simulink model "torque_controller_subsystem_completed_V2_R2019"  (R2019a)
settings: Solver=VariableStepAuto  StartTime=0.0  StopTime=5  RelTol=1e-3
model workspace (MAT data in the model file):
  DCBusVoltage = 24
  K_e = 221.0633
  L_d = 0.003482
  L_q = 0.00456
  Machine_Temperature = 25
  N = 9
  Peak_Current_String = 'Peak Current = 6.000000'
  PhaseAdvancesPerCycle = 36
  Phase_Advance_String = 'PhaseAdvance = 180.000000'
  PointsPerCycle = 36
  Rload = 1000000
  Rs = 0.624570538244
  Shaft_Speed = 27
  MCOS : class17 (value not decoded)
  MCOS : class17 (value not decoded)
  angleVec = [0 1.11111111111 2.22222222222 3.33333333333 4.44444444444 5.55555555556 6.66666666667 7.77777777778 8.88888888889 10 11.1111111111 12.2222222222 ... (37 elements, 1x37)]
  dq_inductance = 0.008366
  fluxAmat = [5.78758604472e-05 -0.00245230641441 -0.00496086974489 -0.00746825845512 -0.00997085180846 -0.0124701917234 -0.0149650380151 -0.0174527751443 -0.0199339133996 -0.0224017046643 -0.0248570910938 -0.0273006981398 ... (16428 elements, 12x37x37)]
  fluxD = 0.129208614948
  fluxDmat = [0.129332720835 0.129331856309 0.129330386347 0.129326055027 0.129320008491 0.129311398581 0.12929964601 0.129284600324 0.129267743431 0.129250546721 0.129230887735 0.129208614948 ... (16428 elements, 12x37x37)]
  fluxQ = -0.0273006981398
  fluxQmat = [5.78758604472e-05 -0.00245230641441 -0.00496086974489 -0.00746825845512 -0.00997085180846 -0.0124701917234 -0.0149650380151 -0.0174527751443 -0.0199339133996 -0.0224017046643 -0.0248570910938 -0.0273006981398 ... (16428 elements, 12x37x37)]
  fluxes = [-0.0273006981398; -0.0982475938625; 0.125548292002]
  funcresult = 0
  gammaVec = [-180 -170 -160 -150 -140 -130 -120 -110 -100 -90 -80 -70 ... (37 elements, 1x37)]
  i = 12
  invP = [-2.44929359829e-16  1; -0.866025403784  -0.5; 0.866025403784  -0.5]
  j = 37
  m = 37
  magVec = [0 0.545454545455 1.09090909091 1.63636363636 2.18181818182 2.72727272727 3.27272727273 3.81818181818 4.36363636364 4.90909090909 5.45454545455 6]
  nGamma = 37
  nMag = 12
  nX = 37
  poleNumber = 18
  pole_pairs = 9
  res1 = 0
  res2 = 0
  res3 = 0
  resistance_per_phase = 0.6246
  torque = -10.6713070894
  torqueMat = [-0.000127780443833 -0.972425785337 -1.94471415001 -2.91686171491 -3.8887574387 -4.86000619896 -5.83073162472 -6.80075888771 -7.77012767412 -8.7384579087 -9.70556312381 -10.6713070894 ... (16428 elements, 12x37x37)]
  torque_constant = 1.7505
  x1 = 360
  x2 = 360
  x3 = 360
  xe = 6.28318530718
  xlabel_string = 'Rotor angle (electrical °)'
  ylabel_string = 'Phase advance (°)'
libraries: fl_lib x12, nesl_utility x12, ee_lib x8, eeTransforms x3, simulink x2, powerlib_meascontrol x1
(part 2 of 2)

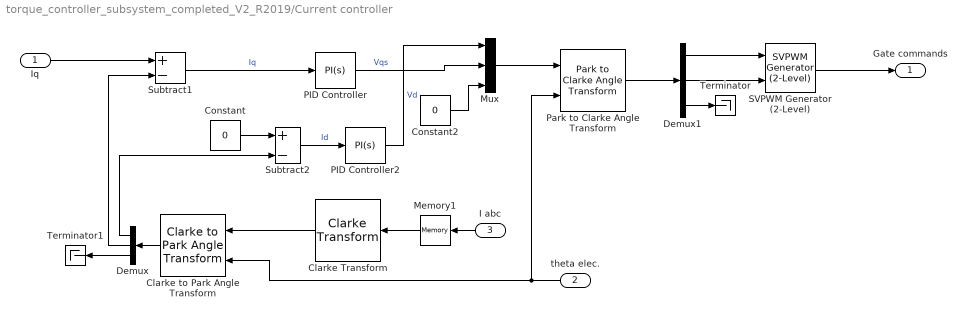
== system torque_controller_subsystem_completed_V2_R2019/Current controller ==
  Iq : Inport
  theta elec. : Inport  Port=2
  I abc : Inport  Port=3
  Clarke Transform : eeTransforms/Clarke Transform  PowerInvariant=off
      settings: SourceProductBaseCode=PS
  Clarke to Park Angle Transform : eeTransforms/Clarke to Park Angle Transform  AxisAlignment=D-axis
      settings: SourceProductBaseCode=PS
  Constant : Constant  Value=0
  Constant2 : Constant  Value=0
  Demux : Demux  Outputs=3
  Demux1 : Demux  Outputs=3
  Memory1 : Memory
  Mux : Mux  Inputs=3
  PID Controller : simulink/Continuous/PID Controller  Controller=PI  Form=Parallel  TimeDomain=Continuous-time  SampleTime=-1  IntegratorMethod=Forward Euler  FilterMethod=Forward Euler  ControllerParametersSource=internal  P=0.23449  I=72.7938  D=0  UseFilter=on  N=100  TunerSelectOption=Transfer Function Based (PID Tuner App)  InitialConditionSource=internal  InitialConditionForIntegrator=0  InitialConditionForFilter=0  DifferentiatorICPrevScaledInput=0  ExternalReset=none  TrackingMode=off  Kt=1  LimitOutput=off  UpperSaturationLimit=inf  LowerSaturationLimit=-inf  LinearizeAsGain=on  AntiWindupMode=none  Kb=1  POutMin=[]  POutMax=[]  IOutMin=[]  IOutMax=[]  DOutMin=[]  DOutMax=[]  NOutMin=[]  NOutMax=[]  SumOutMin=[]  SumOutMax=[]  SaturationOutMin=[]  SaturationOutMax=[]  PParamMin=[]  PParamMax=[]  IParamMin=[]  IParamMax=[]  DParamMin=[]  DParamMax=[]  NParamMin=[]  NParamMax=[]  KbParamMin=[]  KbParamMax=[]  KtParamMin=[]  KtParamMax=[]  KbOutMin=[]  KbOutMax=[]  KtOutMin=[]  KtOutMax=[]  IntegratorOutMin=[]  IntegratorOutMax=[]  FilterOutMin=[]  FilterOutMax=[]  SumI1OutMin=[]  SumI1OutMax=[]  SumI2OutMin=[]  SumI2OutMax=[]  SumI3OutMin=[]  SumI3OutMax=[]  SumI4OutMin=[]  SumI4OutMax=[]  SumDOutMin=[]  SumDOutMax=[]  DifferentiatorOutMin=[]  DifferentiatorOutMax=[]  FilterDiffOutCoefMin=[]  FilterDiffOutCoefMax=[]  ReciprocalOutMin=[]  ReciprocalOutMax=[]  SumDenOutMin=[]  SumDenOutMax=[]  SumNumOutMin=[]  SumNumOutMax=[]  DivideOutMin=[]  DivideOutMax=[]  IntegratorContinuousStateAttributes=''  IntegratorStateMustResolveToSignalObject=off  IntegratorRTWStateStorageClass=Auto  FilterContinuousStateAttributes=''  FilterStateMustResolveToSignalObject=off  FilterRTWStateStorageClass=Auto  ParallelPVariant=InternalParameters  IdealPVariant=Disabled  IVariant=InternalParameters  DVariant=Disabled  IntegratorVariant=Continuous  SatVariant=Disabled  AWVariant=Passthrough  PCopyVariant=Disabled  TRVariant=Disabled  FdbkBlocksVariant=Forward  IdealPFdbkVariant=Disabled  SatFdbkVariant=Disabled  DerivativeFilterVariant=Disabled  NVariant=Disabled  NCopyVariant=Disabled_SignalSpec  FilterICVariant=Disabled  IntegratorICVariant=InternalICs  ExternalResetVariant=Disabled  TRSumVariant=Passthrough  SumFdbkVariant=Disabled  SumVariant=Sum_PI
  PID Controller2 : simulink/Continuous/PID Controller  Controller=PI  Form=Parallel  TimeDomain=Continuous-time  SampleTime=-1  IntegratorMethod=Forward Euler  FilterMethod=Forward Euler  ControllerParametersSource=internal  P=0.17425  I=69.1084  D=0  UseFilter=on  N=100  TunerSelectOption=Transfer Function Based (PID Tuner App)  InitialConditionSource=internal  InitialConditionForIntegrator=0  InitialConditionForFilter=0  DifferentiatorICPrevScaledInput=0  ExternalReset=none  TrackingMode=off  Kt=1  LimitOutput=off  UpperSaturationLimit=inf  LowerSaturationLimit=-inf  LinearizeAsGain=on  AntiWindupMode=none  Kb=1  POutMin=[]  POutMax=[]  IOutMin=[]  IOutMax=[]  DOutMin=[]  DOutMax=[]  NOutMin=[]  NOutMax=[]  SumOutMin=[]  SumOutMax=[]  SaturationOutMin=[]  SaturationOutMax=[]  PParamMin=[]  PParamMax=[]  IParamMin=[]  IParamMax=[]  DParamMin=[]  DParamMax=[]  NParamMin=[]  NParamMax=[]  KbParamMin=[]  KbParamMax=[]  KtParamMin=[]  KtParamMax=[]  KbOutMin=[]  KbOutMax=[]  KtOutMin=[]  KtOutMax=[]  IntegratorOutMin=[]  IntegratorOutMax=[]  FilterOutMin=[]  FilterOutMax=[]  SumI1OutMin=[]  SumI1OutMax=[]  SumI2OutMin=[]  SumI2OutMax=[]  SumI3OutMin=[]  SumI3OutMax=[]  SumI4OutMin=[]  SumI4OutMax=[]  SumDOutMin=[]  SumDOutMax=[]  DifferentiatorOutMin=[]  DifferentiatorOutMax=[]  FilterDiffOutCoefMin=[]  FilterDiffOutCoefMax=[]  ReciprocalOutMin=[]  ReciprocalOutMax=[]  SumDenOutMin=[]  SumDenOutMax=[]  SumNumOutMin=[]  SumNumOutMax=[]  DivideOutMin=[]  DivideOutMax=[]  IntegratorContinuousStateAttributes=''  IntegratorStateMustResolveToSignalObject=off  IntegratorRTWStateStorageClass=Auto  FilterContinuousStateAttributes=''  FilterStateMustResolveToSignalObject=off  FilterRTWStateStorageClass=Auto  ParallelPVariant=InternalParameters  IdealPVariant=Disabled  IVariant=InternalParameters  DVariant=Disabled  IntegratorVariant=Continuous  SatVariant=Disabled  AWVariant=Passthrough  PCopyVariant=Disabled  TRVariant=Disabled  FdbkBlocksVariant=Forward  IdealPFdbkVariant=Disabled  SatFdbkVariant=Disabled  DerivativeFilterVariant=Disabled  NVariant=Disabled  NCopyVariant=Disabled_SignalSpec  FilterICVariant=Disabled  IntegratorICVariant=InternalICs  ExternalResetVariant=Disabled  TRSumVariant=Passthrough  SumFdbkVariant=Disabled  SumVariant=Sum_PI
  Park to Clarke Angle Transform : eeTransforms/Park to Clarke Angle Transform  AxisAlignment=D-axis
      settings: SourceProductBaseCode=PS
  SVPWM Generator (2-Level) : powerlib_meascontrol/Pulse & Signal Generators/SVPWM Generator (2-Level)  InputType=alpha-beta components  SwitchingPattern=Pattern #1  Fc=2000  ParUref=[0.8 -30 50]  Ts=0
      settings: SourceProductBaseCode=PS
  Subtract1 : Sum  Inputs=+-
  Subtract2 : Sum  Inputs=+-
  Terminator : Terminator
  Terminator1 : Terminator
  Gate commands : Outport
  wires:
  theta elec./1 -> Clarke to Park Angle Transform/2, Park to Clarke Angle Transform/2
  Subtract1/1 -> PID Controller/1  "Iq"
  Demux1/1 -> SVPWM Generator (2-Level)/1
  Mux/1 -> Park to Clarke Angle Transform/1
  PID Controller/1 -> Mux/2  "Vqs"
  Demux1/2 -> SVPWM Generator (2-Level)/2
  Clarke Transform/1 -> Clarke to Park Angle Transform/1
  Subtract2/1 -> PID Controller2/1  "Id"
  Demux/1 -> Subtract2/2
  Clarke to Park Angle Transform/1 -> Demux/1
  Demux1/3 -> Terminator/1
  Demux/2 -> Subtract1/2
  Constant2/1 -> Mux/3
  Demux/3 -> Terminator1/1
  Park to Clarke Angle Transform/1 -> Demux1/1
  Constant/1 -> Subtract2/1
  Memory1/1 -> Clarke Transform/1
  PID Controller2/1 -> Mux/1  "Vd"
  SVPWM Generator (2-Level)/1 -> Gate commands/1
  Iq/1 -> Subtract1/1
  I abc/1 -> Memory1/1

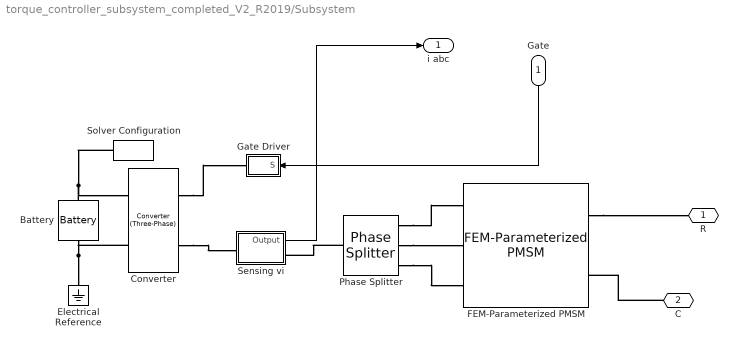
== system torque_controller_subsystem_completed_V2_R2019/Subsystem ==
  Gate : Inport
  Battery : ee_lib/Sources/Battery  Vnom=24 V  R1=2 Ohm  prm_AH=1  AH=50 hr*A  V1=11.5 V  AH1=25 hr*A  prm_R2=1  R2=2000 Ohm  prm_dyn=1  Rp1=0.005 Ohm  tau1=30 s  Rp2=0.005 Ohm  tau2=30 s  Rp3=0.005 Ohm  tau3=30 s  Rp4=0.005 Ohm  tau4=30 s  Rp5=0.005 Ohm  tau5=30 s  prm_fade=1  N_fade=100  AH_fade=45 hr*A  R1_fade=2.02 Ohm  V1_fade=10.35 V  i_specify=off  i_priority=None  i=0 A  i_nominal_specify=off  i_nominal_unit=A  i_nominal_value=1  v_specify=off  v_priority=None  v=0 V  v_nominal_specify=off  v_nominal_unit=V  v_nominal_value=1  charge_specify=off  charge_priority=High  charge=50 hr*A  charge_nominal_specify=off  charge_nominal_unit=hr*A  charge_nominal_value=1  num_cycles_specify=off  num_cycles_priority=High  num_cycles=0  num_cycles_nominal_specify=off  num_cycles_nominal_unit=1  num_cycles_nominal_value=1  thermal_mass=30000 J/K  Tmeas=298.15 K  Vnom_T2=12 V  R1_T2=2.2 Ohm  V1_T2=11.4 V  R2_T2=2200 Ohm  Rp1_T2=0.005 Ohm  tau1_T2=30 s  Rp2_T2=0.005 Ohm  tau2_T2=30 s  Rp3_T2=0.005 Ohm  tau3_T2=30 s  Rp4_T2=0.005 Ohm  tau4_T2=30 s  Rp5_T2=0.005 Ohm  tau5_T2=30 s  Tmeas2=273.15 K  temperature_specify=off  temperature_priority=High  temperature=298.15 K  temperature_nominal_specify=off  temperature_nominal_unit=K  temperature_nominal_value=1
  Converter : ee_lib/Semiconductors & Converters/Converters/Converter (Three-Phase)  device_type=ee.enum.converters.switchingdevice.mosfet  Vf=0.8 V  Ron=17.5*10^-3 Ohm  Rds=17.5 * 10^-3 Ohm  Goff=1e-5 1/Ohm  Vth=0.5 V  Vgt=1 V  Vgt_off=-1 V  Ih=1 A  diode_param=ee.enum.converters.protectiondiode.nodynamics  diode_Vf=0.8 V  diode_Ron=0.001 Ohm  diode_Goff=1e-5 1/Ohm  diode_C=50 nF  diode_iRM=-235 A  diode_iF=300 A  diode_idot=-50 A/us  diode_trr_param=ee.enum.converters.diodetrr.trr_factor  diode_trr_factor=3  diode_trr=15 us  diode_Qrr=1.5e+3 s*uA  snubber_type=ee.enum.converters.snubber.exclude  Rs=0.1 Ohm  Cs=1e-7 F
      settings: SourceProductBaseCode=PS
  Electrical Reference : fl_lib/Electrical/Electrical Elements/Electrical Reference
      settings: SourceProductBaseCode=MT,SS
  FEM-Parameterized PMSM : ee_lib/Electromechanical/Permanent Magnet/FEM-Parameterized PMSM  parameterization=1  winding_type=ee.enum.statorconnection.wye  iVec=[-2, 0, 2] A  xVec=[0, 20, 40, 60] deg  dfluxdiMatrix=0.0002 * ones(3, 4) Wb/A  dfluxdxMatrix=[0, -.16, .16, 0; 0, -.16, .16, 0; 0, -.16, .16, 0] Wb/rad  calculate_torque_matrix=1  TorqueMatrix=zeros(3, 3, 3, 4) N*m  idVec1=[-200, 0, 200] A  iqVec1=[-200, 0, 200] A  LdMatrix=0.0002 * ones(3, 3) H  LqMatrix=0.0002 * ones(3, 3) H  PmMatrix=0.1 * ones(3, 3) Wb  N=6  interp_method=simscape.enum.interpolation.linear  Rs=Rs Ohm  Ms=0.00002 H  losses_oc=[0, 0, 0] W  losses_sc=[0, 0, 0] W  f_losses=140 Hz  Isc_losses=95 A  Inertia=0 kg*m^2  lam=0 N*m/(rad/s)  i_d_specify=off  i_d_priority=High  i_d=0 A  i_d_nominal_specify=off  i_d_nominal_unit=A  i_d_nominal_value=1  i_q_specify=off  i_q_priority=High  i_q=0 A  i_q_nominal_specify=off  i_q_nominal_unit=A  i_q_nominal_value=1  torque_specify=off  torque_priority=None  torque=0 N*m  torque_nominal_specify=off  torque_nominal_unit=N*m  torque_nominal_value=1  angular_velocity_specify=on  angular_velocity_priority=High  angular_velocity=0 rpm  angular_velocity_nominal_specify=off  angular_velocity_nominal_unit=rpm  angular_velocity_nominal_value=1  angular_position_specify=on  angular_position_priority=High  angular_position=0 deg  angular_position_nominal_specify=off  angular_position_nominal_unit=deg  angular_position_nominal_value=1  Tmeas=298.15 K  alpha=3.93e-3 1/K  alpha_flux=-0.001 1/K  stator_thermal_mass=100 J/K  stator_initial_temperatures=[298.15, 298.15, 298.15] K  rotor_thermal_mass=200 J/K  rotor_initial_temperature=298.15 K  Rm_percent_rotor=90  Rd_percent_rotor=30  idVec=[-200, 0, 200] A  iqVec=[-200, 0, 200] A  dfluxAdiaMatrix3D=zeros(3, 3, 4) Wb/A  dfluxAdibMatrix3D=zeros(3, 3, 4) Wb/A  dfluxAdicMatrix3D=zeros(3, 3, 4) Wb/A  dfluxAdxMatrix3D=zeros(3, 3, 4) Wb/rad  TorqueMatrix3D=zeros(3, 3, 4) N*m  iaVec=[-200, 0, 200] A  ibVec=[-200, 0, 200] A  icVec=[-200, 0, 200] A  dfluxAdiaMatrix=zeros(3, 3, 3, 4) Wb/A  dfluxAdibMatrix=zeros(3, 3, 3, 4) Wb/A  dfluxAdicMatrix=zeros(3, 3, 3, 4) Wb/A  dfluxAdxMatrix=zeros(3, 3, 3, 4) Wb/rad  param_dq0=2  winding_type_dq0=ee.enum.statorconnection.wye  nPolePairs=N  parks_type=2  idVec2=[-200, 0, 200] A  iqVec2=[-200, 0, 200] A  magVec2=magVec A  betaVec2=gammaVec deg  xVec2=angleVec deg  fluxD_dq0=zeros(3, 3, 7) Wb  fluxQ_dq0=zeros(3, 3, 7) Wb  fluxA_dq0=zeros(3, 3, 7) Wb  Torque_dq0=zeros(3, 3, 7) N*m  fluxD_IBX=fluxDmat Wb  fluxQ_IBX=fluxQmat Wb  fluxA_IBX=fluxAmat Wb  Torque_IBX=torqueMat N*m
      settings: SourceProductName=Electrical  InternalSimscapePortConfiguration="{\"Bottom\":[],\"Left\":[{\"id\":\"a\",\"label\":\"a\",\"type\":\"foundation.electrical.electrical\"},{\"id\":\"b\",\"label\":\"b\",\"type\":\"foundation.electrical.electrical\"},{\"id\":\"c\",\"label\":\"c\",\"type\":\"foundation.electrical.electrical\"}],\"Right\":[{\"id\":\"R\",\"label\":\"R\",\"type\":\"foundation.mechanical.rotational.rotational\"},{\"id\":\"C\",\"label\":\"C\",\"type\":\"foundation.mechanical.rotational.rotational\"}],\"Top\":[]}"
  Gate Driver : Subsystem
  Phase Splitter : ee_lib/Connectors & References/Phase Splitter
      settings: SourceProductBaseCode=PS
  Sensing vi : Subsystem
      mask Display: disp('vi')
  Solver Configuration : nesl_utility/Solver Configuration  PhysicalDomain=network_engine_domain  SubClassName=solver  LeftPortType=input  RightPortType=generic  Tones=[]  Harmonics=[]  SimulateNoise=off  Profile=off  UseLocalSampling=off  EnableSwitchedLinearOptims=on  FrequencyDomain=off  UseCCode=off  RelTol=0.001  AbsTol=1e-06  MinStep=1e-09  ToWorkspace=off  RevertToSquareIcSolve=off  NumHomotopyIterations=100  PhasorMode=off  PhasorModeNumHarmonics=1  DoDC=off  ResidualTolerance=1e-9  UseLocalSolver=on  LocalSolverChoice=NE_BACKWARD_EULER_ADVANCER  LocalSolverSampleTime=5*10^-7  DoFixedCost=on  MaxNonlinIter=4  MaxModeIter=2  LinearAlgebra=auto  EquationFormulation=NE_TIME_EF  DelaysMemoryBudget=1024  AutomaticFiltering=on  FilteringTimeConstant=0.001  PartitionStorageMethod=AS_NEEDED  PartitionMemoryBudget=1024  PartitionMethod=FAST
      settings: SourceProductBaseCode=MT,SS
  R : PMIOPort  Side=Right
  C : PMIOPort  Port=2  Side=Right
  i abc : Outport
  wires:
  Sensing vi/1(Output) -> i abc/1
  Gate/1 -> Gate Driver/1(S)
  connections:
  Phase Splitter/RConn3 -- FEM-Parameterized PMSM/LConn3
  Converter/LConn1 -- Gate Driver/RConn1
  Converter/RConn2 -- Battery/RConn1 -- Electrical Reference/LConn1
  Phase Splitter/LConn1 -- Sensing vi/RConn1
  Converter/LConn2 -- Sensing vi/LConn1
  Solver Configuration/RConn1 -- Battery/LConn1 -- Converter/RConn1
  Phase Splitter/RConn1 -- FEM-Parameterized PMSM/LConn1
  Phase Splitter/RConn2 -- FEM-Parameterized PMSM/LConn2
  C/RConn1 -- FEM-Parameterized PMSM/RConn2
  FEM-Parameterized PMSM/RConn1 -- R/RConn1

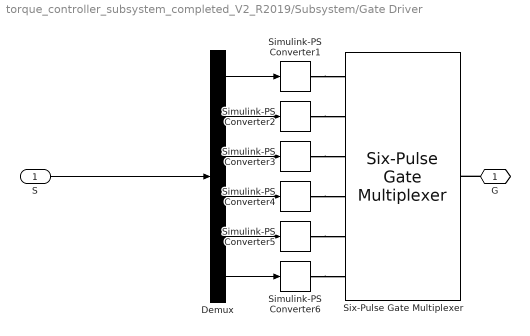
== system torque_controller_subsystem_completed_V2_R2019/Subsystem/Gate Driver ==
  S : Inport
  Demux : Demux  Outputs=6
  Simulink-PS Converter{1..6} (6 alike) : nesl_utility/Simulink-PS Converter  PhysicalDomain=network_engine_domain  SubClassName=ps_input  LeftPortType=input  RightPortType=output  PseudoPeriodic=off  Frequencies=[]  NoiseDistribution=none  NoiseParameters=[]  Unit=1  AffineConversion=off  FilteringAndDerivatives=zero  SimscapeFilterOrder=1  InputFilterTimeConstant=0.001  UdotUserProvided=1
      settings: SourceProductBaseCode=MT,SS
  Six-Pulse Gate Multiplexer : ee_lib/Semiconductors & Converters/Converters/Six-Pulse Gate Multiplexer  R=0 Ohm
      settings: SourceProductBaseCode=PS  InternalSimscapePortConfiguration="{\"Bottom\":[],\"Left\":[{\"id\":\"GaH\",\"label\":\"Ga(H)\",\"type\":\"input\"},{\"id\":\"GaL\",\"label\":\"Ga(L)\",\"type\":\"input\"},{\"id\":\"GbH\",\"label\":\"Gb(H)\",\"type\":\"input\"},{\"id\":\"GbL\",\"label\":\"Gb(L)\",\"type\":\"input\"},{\"id\":\"GcH\",\"label\":\"Gc(H)\",\"type\":\"input\"},{\"id\":\"GcL\",\"label\":\"Gc(L)\",\"type\":\"input\"}],\"Right\":[{\"id\":\"p\",\"label\":\"G\",\"type\":\"foundation.electrical.twelve_phase\"}],\"Top\":[]}"
  G : PMIOPort  Side=Right
  wires:
  Demux/1 -> Simulink-PS Converter1/1
  Demux/4 -> Simulink-PS Converter4/1
  Demux/2 -> Simulink-PS Converter2/1
  Demux/3 -> Simulink-PS Converter3/1
  Demux/5 -> Simulink-PS Converter5/1
  Demux/6 -> Simulink-PS Converter6/1
  S/1 -> Demux/1
  connections:
  G/RConn1 -- Six-Pulse Gate Multiplexer/RConn1
  Simulink-PS Converter5/RConn1 -- Six-Pulse Gate Multiplexer/LConn5
  Simulink-PS Converter4/RConn1 -- Six-Pulse Gate Multiplexer/LConn4
  Simulink-PS Converter6/RConn1 -- Six-Pulse Gate Multiplexer/LConn6
  Simulink-PS Converter3/RConn1 -- Six-Pulse Gate Multiplexer/LConn3
  Simulink-PS Converter2/RConn1 -- Six-Pulse Gate Multiplexer/LConn2
  Simulink-PS Converter1/RConn1 -- Six-Pulse Gate Multiplexer/LConn1

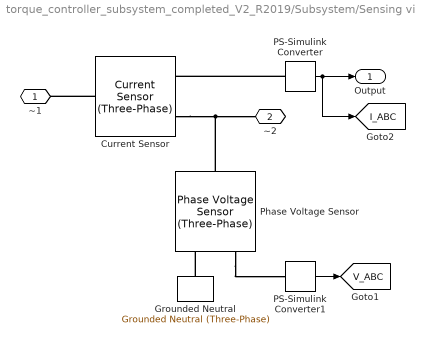
== system torque_controller_subsystem_completed_V2_R2019/Subsystem/Sensing vi ==
  Current Sensor : ee_lib/Sensors & Transducers/Current Sensor (Three-Phase)
  Grounded Neutral : ee_lib/Connectors & References/Grounded Neutral (Three-Phase)
      settings: SourceProductBaseCode=PS
  PS-Simulink Converter : nesl_utility/PS-Simulink Converter  PhysicalDomain=network_engine_domain  SubClassName=ps_output  LeftPortType=input  RightPortType=output  PseudoPeriodic=off  Frequencies=[]  Unit=A  AffineConversion=off
      settings: SourceProductBaseCode=MT,SS
  PS-Simulink Converter1 : nesl_utility/PS-Simulink Converter  PhysicalDomain=network_engine_domain  SubClassName=ps_output  LeftPortType=input  RightPortType=output  PseudoPeriodic=off  Frequencies=[]  Unit=V  AffineConversion=off
      settings: SourceProductBaseCode=MT,SS
  Phase Voltage Sensor : ee_lib/Sensors & Transducers/Phase Voltage Sensor (Three-Phase)
      settings: SourceProductBaseCode=PS
  ~1 : PMIOPort  Side=Left
  ~2 : PMIOPort  Port=2  Side=Right
  Output : Outport
  tag scope: I_ABC=global, V_ABC=global
  wires:
  PS-Simulink Converter1/1 -> [V_ABC]
  PS-Simulink Converter/1 -> [I_ABC], Output/1
  connections:
  Current Sensor/LConn1 -- ~1/RConn1
  PS-Simulink Converter/LConn1 -- Current Sensor/RConn1
  Current Sensor/RConn2 -- Phase Voltage Sensor/LConn1 -- ~2/RConn1
  Phase Voltage Sensor/RConn1 -- PS-Simulink Converter1/LConn1
  Grounded Neutral/LConn1 -- Phase Voltage Sensor/RConn2
